simulink model "Ras2_og_1"  (R2014b)
settings: Solver=ode45  StartTime=0.0  StopTime=10.0  RelTol=1e-3
libraries: simulink x1
settings Model: Creator=kristofer  LastModifiedBy=kristofer

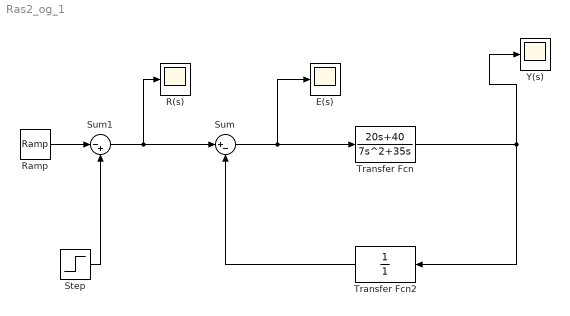
== system Ras2_og_1 ==
  E(s) : Scope
      settings: SaveName=ScopeData2
  R(s) : Scope
  Ramp : simulink/Sources/Ramp  slope=1  start=0  X0=0
  Step : Step  Time=0  SampleTime=0
  Sum : Sum  Inputs=|+-
  Sum1 : Sum  Inputs=|-+
  Transfer Fcn : TransferFcn  Numerator=[20 40]  Denominator=[7 35 0]
  Transfer Fcn2 : TransferFcn  Denominator=[0 1]
  Y(s) : Scope
  wires:
  Transfer Fcn/1 -> Transfer Fcn2/1, Y(s)/1
  Sum/1 -> Transfer Fcn/1, E(s)/1
  Transfer Fcn2/1 -> Sum/2
  Ramp/1 -> Sum1/1
  Sum1/1 -> R(s)/1, Sum/1
  Step/1 -> Sum1/2
